simulink model "torch_pos_with_sensors_tuning(1)"  (R2024a)
settings: Solver=FixedStepAuto  StartTime=0.0  StopTime=50  FixedStep=framePeriod_s  RelTol=1e-3
undefined symbols (not defined in the file): Aircraft, DiscIntNeverNeededParam, framePeriod_s, frameRate_hz, magnitude
libraries: simulink x37, slpidlib x10, simulink_extras x2, dspmathops x1
(part 2 of 4)

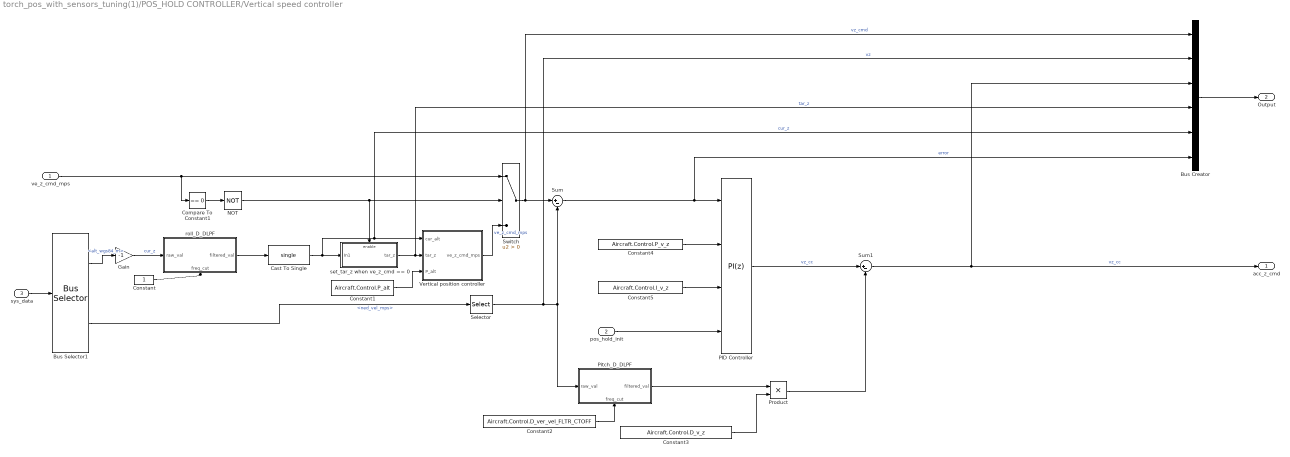
== system torch_pos_with_sensors_tuning(1)/POS_HOLD CONTROLLER/Vertical speed controller ==
  ve_z_cmd_mps : Inport
  pos_hold_init : Inport  Port=2
  sys_data : Inport  Port=3
  Bus Creator : BusCreator  Inputs=6
  Bus Selector1 : BusSelector  OutputSignals=Sensor Data.ext_gnss1.alt_wgs84_m,StateEstData.bfs_ins.ned_vel_mps
  Cast To Single : DataTypeConversion  OutDataTypeStr=single  SaturateOnIntegerOverflow=off  RndMeth=Floor
  Compare To Constant1 : simulink/Logic and Bit Operations/Compare To Constant  relop===  const=0  OutDataTypeStr=boolean
  Constant : Constant  OutDataTypeStr=single
  Constant1 : Constant  Value=Aircraft.Control.P_alt  OutDataTypeStr=single
  Constant2 : Constant  Value=Aircraft.Control.D_ver_vel_FLTR_CTOFF  OutDataTypeStr=single
  Constant3 : Constant  Value=Aircraft.Control.D_v_z  OutDataTypeStr=single
  Constant4 : Constant  Value=Aircraft.Control.P_v_z  OutDataTypeStr=single
  Constant5 : Constant  Value=Aircraft.Control.I_v_z  OutDataTypeStr=single
  Gain : Gain  Gain=-1
  NOT : Logic  Operator=NOT  IconShape=distinctive  AllPortsSameDT=off  OutDataTypeStr=boolean
  PID Controller : slpidlib/PID Controller  Controller=PI  Form=Parallel  TimeDomain=Discrete-time  UseExternalTs=off  SampleTime=framePeriod_s  IntegratorMethod=Forward Euler  FilterMethod=Forward Euler  ControllerParametersSource=external  P=0  I=0  UseKiTs=off  D=0  UseExternalDerivativeSource=off  N=100  UseFilter=off  TunerSelectOption=Frequency Response Based  InitialConditionSource=internal  InitialConditionForIntegrator=0  InitialConditionForFilter=0  DifferentiatorICPrevScaledInput=0  ExternalReset=either  TrackingMode=off  Kt=1  LimitOutput=on  SatLimitsSource=internal  UpperSaturationLimit=1  LowerSaturationLimit=-1  LinearizeAsGain=on  AntiWindupMode=clamping  Kb=1  LimitIntegrator=off  UpperIntegratorSaturationLimit=inf  LowerIntegratorSaturationLimit=-inf  POutMin=[]  POutMax=[]  IOutMin=[]  IOutMax=[]  DOutMin=[]  DOutMax=[]  NOutMin=[]  NOutMax=[]  SumOutMin=[]  SumOutMax=[]  SaturationOutMin=[]  SaturationOutMax=[]  PParamMin=[]  PParamMax=[]  IParamMin=[]  IParamMax=[]  DParamMin=[]  DParamMax=[]  NParamMin=[]  NParamMax=[]  KbParamMin=[]  KbParamMax=[]  KtParamMin=[]  KtParamMax=[]  KbOutMin=[]  KbOutMax=[]  KtOutMin=[]  KtOutMax=[]  IntegratorOutMin=[]  IntegratorOutMax=[]  FilterOutMin=[]  FilterOutMax=[]  SumI1OutMin=[]  SumI1OutMax=[]  SumI2OutMin=[]  SumI2OutMax=[]  SumI3OutMin=[]  SumI3OutMax=[]  SumI4OutMin=[]  SumI4OutMax=[]  SumDOutMin=[]  SumDOutMax=[]  DifferentiatorOutMin=[]  DifferentiatorOutMax=[]  FilterDiffOutCoefMin=[]  FilterDiffOutCoefMax=[]  ReciprocalOutMin=[]  ReciprocalOutMax=[]  SumDenOutMin=[]  SumDenOutMax=[]  SumNumOutMin=[]  SumNumOutMax=[]  DivideOutMin=[]  DivideOutMax=[]  UdiffTsProdOutMin=[]  UdiffTsProdOutMax=[]  NTsProdOutMin=[]  NTsProdOutMax=[]  UintegralTsProdOutMin=[]  UintegralTsProdOutMax=[]  UngainTsProdOutMin=[]  UngainTsProdOutMax=[]  ClampingZeroOutDataTypeStr=Inherit: Inherit via back propagation  ClampingZeroOutMin=[]  ClampingZeroOutMax=[]  FilterDenConstantOutDataTypeStr=Inherit: Inherit via back propagation  FilterDenConstantOutMin=[]  FilterDenConstantOutMax=[]  PCopyOutDataTypeStr=Inherit: Inherit via back propagation  PCopyOutMin=[]  PCopyOutMax=[]  NCopyOutDataTypeStr=Inherit: Inherit via back propagation  NCopyOutMin=[]  NCopyOutMax=[]  IntegratorContinuousStateAttributes=''  IntegratorStateMustResolveToSignalObject=off  IntegratorRTWStateStorageClass=Auto  FilterContinuousStateAttributes=''  FilterStateMustResolveToSignalObject=off  FilterRTWStateStorageClass=Auto  ParallelPVariant=ExternalParameters  IdealPVariant=Disabled  IVariant=ExternalParameters  DVariant=Disabled  IntegratorVariant=Discrete  SatVariant=Enabled  AWVariant=DiscClampingParallel  PCopyVariant=Disabled  TRVariant=Disabled  FdbkBlocksVariant=Forward  IdealPFdbkVariant=Disabled  SatFdbkVariant=Disabled  DerivativeFilterVariant=Disabled  NVariant=Disabled  NCopyVariant=Disabled_SignalSpec  FilterICVariant=Disabled  IntegratorICVariant=InternalICs  ExternalResetVariant=ExternalReset  TRSumVariant=Passthrough  SumFdbkVariant=Disabled  SumVariant=Sum_PI  TsampFilterVariant=InternalTs  TsampNgainVariant=Passthrough  TsampIntegralVariant=Disabled_SignalSpec  ExternalSaturationOutDataTypeStr=Inherit: Same as second input  DerivativeSourceVariant=Disabled
  Pitch_D_DLPF : Subsystem
      settings: PortSchema="{\"entries\":[{\"content\":{\"sides\":[{\"content\":{\"connectorIds\":[\"In1\"]},\"type\":\"ConnectorPlacement.EquallySpacedRectSide\",\"uuid\":\"20236834-aeb3-4c5b-bb2e-f84447e752b5\"},{\"content\":{\"connectorIds\":[\"Out1\"],\"side\":\"RIGHT\"},\"type\":\"ConnectorPlacement.EquallySpacedRectSide\",\"uuid\":\"d668f9a1-a3df-4207-8bf1-99fb838e59b2\"},{\"content\":{\"connectorIds\":[],\"side\":\"TOP\"},\"type\":\"ConnectorPlacement.EquallySpacedRectSide\",\"uuid\":\"66cceb06-f4bc-4278-b965-2427292e46df\"},{\"content\":{\"connectorIds\":[\"In2\"],\"side\":\"BOTTOM\"},\"type\":\"ConnectorPlacement.EquallySpacedRectSide\",\"uuid\":\"7d08bc25-8e2d-44c6-8f94-b04e75c70268\"}]},\"type\":\"ConnectorPlacement.EquallySpacedConnector\",\"uuid\":\"3dc29a9a-e794-478d-b7df-452e6c2d3f66\"}],\"packageUris\":[\"http://schema.mathworks.com/mf0/Connector/R2020b\"],\"version\":\"1.0\"}"
  Product : Product
  Selector : Selector  InputPortWidth=3  IndexOptions=Index vector (dialog)  Indices=[3]  OutputSizes=1
  Sum : Sum  Inputs=|+-
  Sum1 : Sum  Inputs=|+-
  Switch : Switch  Criteria=u2 > Threshold  SaturateOnIntegerOverflow=off  InputSameDT=off
  Vertical position controller : Subsystem
  roll_D_DLPF : Subsystem
      settings: PortSchema="{\"entries\":[{\"content\":{\"sides\":[{\"content\":{\"connectorIds\":[\"In1\"]},\"type\":\"ConnectorPlacement.EquallySpacedRectSide\",\"uuid\":\"20236834-aeb3-4c5b-bb2e-f84447e752b5\"},{\"content\":{\"connectorIds\":[\"Out1\"],\"side\":\"RIGHT\"},\"type\":\"ConnectorPlacement.EquallySpacedRectSide\",\"uuid\":\"d668f9a1-a3df-4207-8bf1-99fb838e59b2\"},{\"content\":{\"connectorIds\":[],\"side\":\"TOP\"},\"type\":\"ConnectorPlacement.EquallySpacedRectSide\",\"uuid\":\"66cceb06-f4bc-4278-b965-2427292e46df\"},{\"content\":{\"connectorIds\":[\"In2\"],\"side\":\"BOTTOM\"},\"type\":\"ConnectorPlacement.EquallySpacedRectSide\",\"uuid\":\"8fdaac6a-cb03-4bd4-87bb-7bafd10bc297\"}]},\"type\":\"ConnectorPlacement.EquallySpacedConnector\",\"uuid\":\"3dc29a9a-e794-478d-b7df-452e6c2d3f66\"}],\"packageUris\":[\"http://schema.mathworks.com/mf0/Connector/R2020b\"],\"version\":\"1.0\"}"
  set_tar_z when ve_z_cmd == 0 : Subsystem  TreatAsAtomicUnit=on
  acc_z_cmd : Outport
  Output : Outport  Port=2
  wires:
  Constant4/1 -> PID Controller/2
  Bus Selector1/2 -> Selector/1  "<ned_vel_mps>"
  sys_data/1 -> Bus Selector1/1
  Pitch_D_DLPF/1(filtered_val) -> Product/1
  Selector/1 -> Bus Creator/2, Sum/2, Pitch_D_DLPF/1(raw_val)  "vz"
  Constant3/1 -> Product/2
  Product/1 -> Sum1/2
  ve_z_cmd_mps/1 -> Compare To Constant1/1, Switch/1
  Compare To Constant1/1 -> NOT/1
  Switch/1 -> Bus Creator/1, Sum/1  "vz_cmd"
  set_tar_z when ve_z_cmd == 0/1(tar_z) -> Bus Creator/4, Vertical position controller/2(tar_z)  "tar_z"
  pos_hold_init/1 -> PID Controller/4
  Constant2/1 -> Pitch_D_DLPF/2(freq_cut)
  Constant1/1 -> Vertical position controller/3(P_alt)
  Bus Creator/1 -> Output/1
  Cast To Single/1 -> Bus Creator/5, Vertical position controller/1(cur_alt), set_tar_z when ve_z_cmd == 0/1(In1)  "cur_z"
  Sum/1 -> Bus Creator/6, PID Controller/1  "error"
  Sum1/1 -> acc_z_cmd/1, Bus Creator/3  "vz_cc"
  PID Controller/1 -> Sum1/1  "vz_cc"
  Constant5/1 -> PID Controller/3
  Vertical position controller/1(ve_z_cmd_mps) -> Switch/3  "ve_z_cmd_mps"
  NOT/1 -> Switch/2, set_tar_z when ve_z_cmd == 0/Enable
  Bus Selector1/1 -> Gain/1  "<alt_wgs84_m>"
  Gain/1 -> roll_D_DLPF/1(raw_val)  "cur_z"
  roll_D_DLPF/1(filtered_val) -> Cast To Single/1
  Constant/1 -> roll_D_DLPF/2(freq_cut)

== system torch_pos_with_sensors_tuning(1)/Stab_input_conversion/remap from min_spin to max ==
  raw_in : Inport
  Constant4 : Constant  Value=0  OutDataTypeStr=single
  Constant5 : Constant  Value=Aircraft.Control.motor_spin_min  OutDataTypeStr=single
  Constant6 : Constant  Value=0.8  OutDataTypeStr=single
  Constant7 : Constant  OutDataTypeStr=single
  remap1 : MATLAB Function  TreatAsAtomicUnit=on
  norm_out : Outport
  wires:
  Constant6/1 -> remap1/5(out_max)
  Constant5/1 -> remap1/4(out_min)
  remap1/1(norm_out) -> norm_out/1
  Constant4/1 -> remap1/2(in_min)
  Constant7/1 -> remap1/3(in_max)
  raw_in/1 -> remap1/1(raw_in)

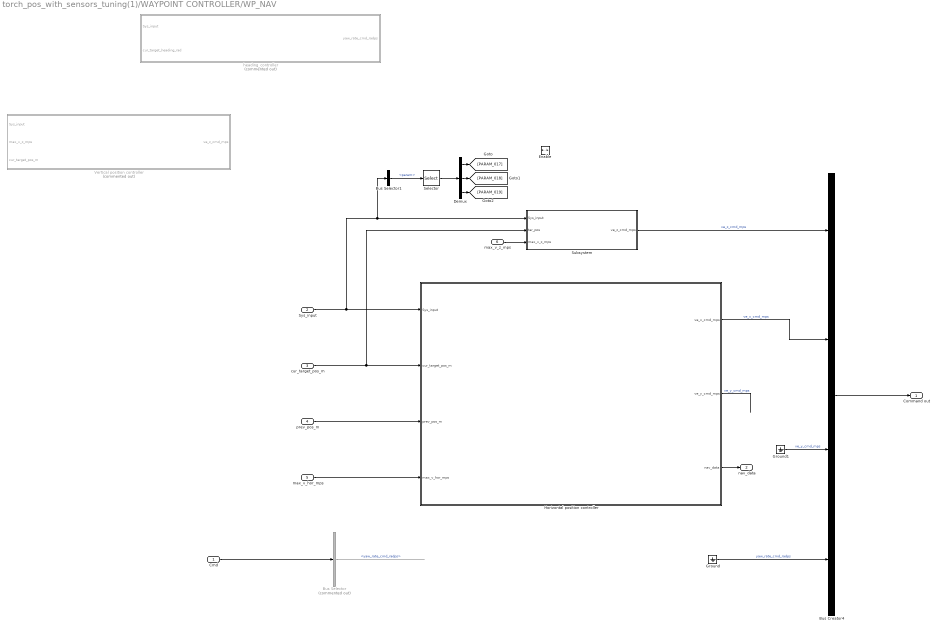
== system torch_pos_with_sensors_tuning(1)/WAYPOINT CONTROLLER/WP_NAV ==
  Cmd : Inport
  Sys_input : Inport  Port=2
  cur_target_pos_m : Inport  Port=3
  prev_pos_m : Inport  Port=4
  max_v_hor_mps : Inport  Port=5
  max_v_z_mps : Inport  Port=6
  Enable : EnablePort
  Bus Creator4 : BusCreator  Inputs=4
  Bus Selector : BusSelector  Commented=on  OutputSignals=yaw_rate_cmd_radps
  Bus Selector1 : BusSelector  OutputSignals=Telemetry Data.param
  Demux : Demux  Outputs=3
  Ground : Ground
  Ground1 : Ground
  Horizontal position controller : Subsystem
  Selector : Selector  IndexMode=Zero-based  InputPortWidth=24  IndexOptions=Index vector (dialog)  Indices=[17 18 19]  OutputSizes=1
  Subsystem : Subsystem
  Vertical position controller : Subsystem  Commented=on
  heading_controller : Subsystem  Commented=on
  Command out : Outport
  nav_data : Outport  Port=2
  wires:
  Bus Creator4/1 -> Command out/1
  Horizontal position controller/1(ve_x_cmd_mps) -> Bus Creator4/2  "ve_x_cmd_mps"
  Horizontal position controller/2(ve_y_cmd_mps) -> ?  "ve_y_cmd_mps"
  Sys_input/1 -> Horizontal position controller/1(Sys_input), Bus Selector1/1, Subsystem/1(Sys_input)
  cur_target_pos_m/1 -> Subsystem/2(tar_pos), Horizontal position controller/2(cur_target_pos_m)
  Cmd/1 -> Bus Selector/1
  Bus Selector/1 -> ?  "<yaw_rate_cmd_radps>"
  prev_pos_m/1 -> Horizontal position controller/3(prev_pos_m)
  max_v_hor_mps/1 -> Horizontal position controller/4(max_v_hor_mps)
  Subsystem/1(ve_z_cmd_mps) -> Bus Creator4/1  "ve_z_cmd_mps"
  max_v_z_mps/1 -> Subsystem/3(max_v_z_mps)
  Horizontal position controller/3(nav_data) -> nav_data/1
  Ground/1 -> Bus Creator4/4  "yaw_rate_cmd_radps"
  Ground1/1 -> Bus Creator4/3  "ve_y_cmd_mps"
  Selector/1 -> Demux/1
  Demux/1 -> [PARAM_017]
  Demux/2 -> [PARAM_018]
  Demux/3 -> [PARAM_019]
  Bus Selector1/1 -> Selector/1  "<param>"

== system torch_pos_with_sensors_tuning(1)/WAYPOINT CONTROLLER/capture rising edge ==
  <current_waypoint> : Inport
  Detect Change1 : simulink/Logic and Bit Operations/Detect Change  vinit=-1  OutDataTypeStr=boolean
  Detect Rise Positive : simulink/Logic and Bit Operations/Detect Rise Positive  Commented=through  vinit=0  OutDataTypeStr=boolean
  enable : Outport
  wires:
  <current_waypoint>/1 -> Detect Change1/1
  Detect Rise Positive/1 -> enable/1
  Detect Change1/1 -> Detect Rise Positive/1

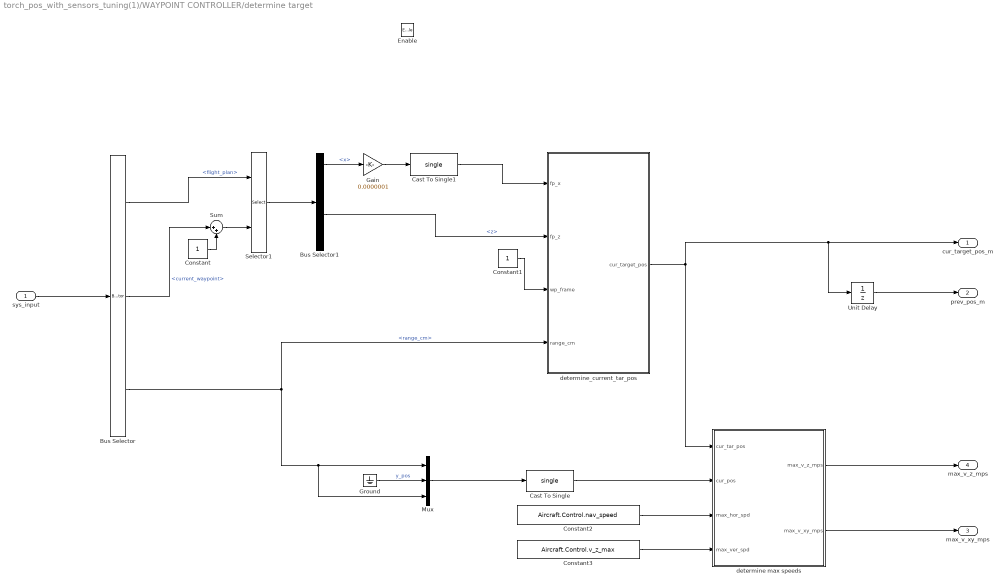
== system torch_pos_with_sensors_tuning(1)/WAYPOINT CONTROLLER/determine target ==
  sys_input : Inport
  Enable : EnablePort  PropagateVarSize=During execution
  Bus Selector : BusSelector  OutputSignals=Telemetry Data.flight_plan,Telemetry Data.current_waypoint,Sensor Data.tfmini.range_cm
  Bus Selector1 : BusSelector  OutputSignals=x,y,z,frame
  Cast To Single : DataTypeConversion  OutDataTypeStr=single  SaturateOnIntegerOverflow=off  RndMeth=Floor
  Cast To Single1 : DataTypeConversion  OutDataTypeStr=single  SaturateOnIntegerOverflow=off  RndMeth=Floor
  Constant : Constant  OutDataTypeStr=int16
  Constant1 : Constant  OutDataTypeStr=uint8
  Constant2 : Constant  Value=Aircraft.Control.nav_speed  OutDataTypeStr=single
  Constant3 : Constant  Value=Aircraft.Control.v_z_max  OutDataTypeStr=single
  Gain : Gain  Gain=0.0000001  OutDataTypeStr=double
  Ground : Ground
  Mux : Mux  Inputs=3
  Selector1 : Selector  IndexMode=Zero-based  InputPortWidth=500  IndexOptions=Index vector (port)  Indices=[1 3]  OutputSizes=1
  Sum : Sum  Inputs=|++
  Unit Delay : UnitDelay  InitialCondition=[0 0 0]  SampleTime=-1  HasFrameUpgradeWarning=on
  determine max speeds : MATLAB Function  TreatAsAtomicUnit=on
  determine_current_tar_pos : MATLAB Function  TreatAsAtomicUnit=on
  cur_target_pos_m : Outport
  prev_pos_m : Outport  Port=2
  max_v_xy_mps : Outport  Port=3
  max_v_z_mps : Outport  Port=4
  wires:
  sys_input/1 -> Bus Selector/1
  Selector1/1 -> Bus Selector1/1
  Bus Selector1/3 -> determine_current_tar_pos/2(fp_z)  "<z>"
  Bus Selector1/1 -> Gain/1  "<x>"
  Bus Selector/1 -> Selector1/1  "<flight_plan>"
  Gain/1 -> Cast To Single1/1
  Sum/1 -> Selector1/2
  Constant/1 -> Sum/2
  Constant1/1 -> determine_current_tar_pos/3(wp_frame)
  Unit Delay/1 -> prev_pos_m/1
  determine_current_tar_pos/1(cur_target_pos) -> cur_target_pos_m/1, Unit Delay/1, determine max speeds/1(cur_tar_pos)
  Cast To Single1/1 -> determine_current_tar_pos/1(fp_x)
  Constant2/1 -> determine max speeds/3(max_hor_spd)
  Constant3/1 -> determine max speeds/4(max_ver_spd)
  determine max speeds/1(max_v_z_mps) -> max_v_z_mps/1
  determine max speeds/2(max_v_xy_mps) -> max_v_xy_mps/1
  Bus Selector/3 -> Mux/3, Mux/1, determine_current_tar_pos/4(range_cm)  "<range_cm>"
  Bus Selector/2 -> Sum/1  "<current_waypoint>"
  Mux/1 -> Cast To Single/1
  Ground/1 -> Mux/2  "y_pos"
  Cast To Single/1 -> determine max speeds/2(cur_pos)

== system torch_pos_with_sensors_tuning(1)/WAYPOINT CONTROLLER/wp_completion_check ==
  note: Output wp_reached cmd only when distance between current pos and target pos is less than wp_radius.
  target_pos : Inport
  Sys_input : Inport  Port=2
  Bus Selector : BusSelector  OutputSignals=Sensor Data.tfmini.range_cm
  Constant : Constant  Value=Aircraft.Control.wp_radius  OutDataTypeStr=single
  check_wp_reached : MATLAB Function  TreatAsAtomicUnit=on
  wp_reached : Outport
  wires:
  Sys_input/1 -> Bus Selector/1
  Bus Selector/1 -> check_wp_reached/2(range_cm)  "<range_cm>"
  check_wp_reached/1(reached) -> wp_reached/1
  target_pos/1 -> check_wp_reached/1(target_pos)
  Constant/1 -> check_wp_reached/3(Aircraft_Control_wp_radius)

== system torch_pos_with_sensors_tuning(1)/WAYPOINT CONTROLLER CMD/Throttle Mapper ==
  Throttle : Inport
  Compare To Constant : simulink/Logic and Bit Operations/Compare To Constant  relop=<  const=0  OutDataTypeStr=boolean
  Compare To Constant1 : simulink/Logic and Bit Operations/Compare To Constant  relop=>=  const=0  OutDataTypeStr=boolean
  Constant : Constant  Value=Aircraft.Control.v_z_down_max  OutDataTypeStr=single
  Constant1 : Constant  Value=Aircraft.Control.v_z_up_max  OutDataTypeStr=single
  Double : Constant  Value=2  OutDataTypeStr=single
  Gain : Gain  Gain=-1
  Normalize at Zero : Constant  Value=0.5  OutDataTypeStr=single
  Product : Product  Inputs=3
  Product1 : Product  Inputs=3
  Sum : Sum  Inputs=|+-
  Sum1 : Sum
  v_z_cmd (-1 to 1) : Product
  Relative Velocity : Outport
  wires:
  Throttle/1 -> Sum/1
  Normalize at Zero/1 -> Sum/2
  Double/1 -> v_z_cmd (-1 to 1)/2
  Sum/1 -> v_z_cmd (-1 to 1)/1
  Sum1/1 -> Gain/1
  v_z_cmd (-1 to 1)/1 -> Product1/2, Compare To Constant1/1, Compare To Constant/1, Product/3
  Constant1/1 -> Product1/3
  Compare To Constant1/1 -> Product1/1
  Product/1 -> Sum1/1
  Product1/1 -> Sum1/2
  Constant/1 -> Product/1
  Compare To Constant/1 -> Product/2
  Gain/1 -> Relative Velocity/1

== system torch_pos_with_sensors_tuning(1)/WAYPOINT CONTROLLER CMD/pitch_norm_deadband ==
  raw_sbus_in : Inport
  deadband : Inport  Port=2
  Constant : Constant  Value=0  OutDataTypeStr=single
  Constant1 : Constant  Value=0  OutDataTypeStr=single
  Constant2 : Constant  OutDataTypeStr=single
  Constant3 : Constant  OutDataTypeStr=single
  remap_with_deadband : MATLAB Function  TreatAsAtomicUnit=on
  normalized_out : Outport
  wires:
  deadband/1 -> remap_with_deadband/6(deadband)
  Constant2/1 -> remap_with_deadband/5(out_max)
  Constant1/1 -> remap_with_deadband/4(out_min)
  Constant3/1 -> remap_with_deadband/3(in_max)
  Constant/1 -> remap_with_deadband/2(in_min)
  remap_with_deadband/1(norm_out) -> normalized_out/1
  raw_sbus_in/1 -> remap_with_deadband/1(raw_in)

== system torch_pos_with_sensors_tuning(1)/WAYPOINT CONTROLLER CMD/remap from min_spin to max ==
  raw_in : Inport
  Constant4 : Constant  Value=0  OutDataTypeStr=single
  Constant5 : Constant  Value=Aircraft.Control.motor_spin_min  OutDataTypeStr=single
  Constant6 : Constant  OutDataTypeStr=single
  Constant7 : Constant  OutDataTypeStr=single
  remap1 : MATLAB Function  TreatAsAtomicUnit=on
  norm_out : Outport
  wires:
  Constant6/1 -> remap1/5(out_max)
  Constant5/1 -> remap1/4(out_min)
  remap1/1(norm_out) -> norm_out/1
  Constant4/1 -> remap1/2(in_min)
  Constant7/1 -> remap1/3(in_max)
  raw_in/1 -> remap1/1(raw_in)

== system torch_pos_with_sensors_tuning(1)/cmd to raw pwm1/motor_PWM_denormalize ==
  normalized_input : Inport
  Constant : Constant  Value=0  OutDataTypeStr=single
  Constant1 : Constant  Value=1100  OutDataTypeStr=single
  Constant2 : Constant  Value=1950  OutDataTypeStr=single
  Constant3 : Constant  OutDataTypeStr=single
  remap : MATLAB Function  TreatAsAtomicUnit=on
  raw_output : Outport
  wires:
  Constant2/1 -> remap/5(out_max)
  Constant1/1 -> remap/4(out_min)
  Constant3/1 -> remap/3(in_max)
  Constant/1 -> remap/2(in_min)
  remap/1(raw_out) -> raw_output/1
  normalized_input/1 -> remap/1(norm_in)

== system torch_pos_with_sensors_tuning(1)/command selection/e_stop_norm ==
  raw_sbus_in : Inport
  Constant : Constant  Value=172  OutDataTypeStr=single
  Constant1 : Constant  Value=-1  OutDataTypeStr=single
  Constant2 : Constant  OutDataTypeStr=single
  Constant3 : Constant  Value=1811  OutDataTypeStr=single
  remap : MATLAB Function  TreatAsAtomicUnit=on
  normalized_out : Outport
  wires:
  Constant2/1 -> remap/5(out_max)
  Constant1/1 -> remap/4(out_min)
  Constant3/1 -> remap/3(in_max)
  Constant/1 -> remap/2(in_min)
  remap/1(norm_out) -> normalized_out/1
  raw_sbus_in/1 -> remap/1(raw_in)

== system torch_pos_with_sensors_tuning(1)/command selection/mode_norm ==
  raw_sbus_in : Inport
  Constant : Constant  Value=172  OutDataTypeStr=single
  Constant1 : Constant  Value=0  OutDataTypeStr=single
  Constant2 : Constant  Value=2  OutDataTypeStr=single
  Constant3 : Constant  Value=1811  OutDataTypeStr=single
  remap : MATLAB Function  TreatAsAtomicUnit=on
  normalized_out : Outport
  wires:
  raw_sbus_in/1 -> remap/1(raw_in)
  remap/1(norm_out) -> normalized_out/1
  Constant/1 -> remap/2(in_min)
  Constant3/1 -> remap/3(in_max)
  Constant1/1 -> remap/4(out_min)
  Constant2/1 -> remap/5(out_max)

== system torch_pos_with_sensors_tuning(1)/command selection/mode_norm1 ==
  raw_sbus_in : Inport
  Constant : Constant  Value=172  OutDataTypeStr=single
  Constant1 : Constant  Value=0  OutDataTypeStr=single
  Constant2 : Constant  OutDataTypeStr=single
  Constant3 : Constant  Value=1811  OutDataTypeStr=single
  remap : MATLAB Function  TreatAsAtomicUnit=on
  normalized_out : Outport
  wires:
  Constant2/1 -> remap/5(out_max)
  Constant1/1 -> remap/4(out_min)
  Constant3/1 -> remap/3(in_max)
  Constant/1 -> remap/2(in_min)
  remap/1(norm_out) -> normalized_out/1
  raw_sbus_in/1 -> remap/1(raw_in)

== system torch_pos_with_sensors_tuning(1)/command selection/pitch_norm_deadband ==
  raw_sbus_in : Inport
  deadband : Inport  Port=2
  Constant : Constant  Value=172  OutDataTypeStr=single
  Constant1 : Constant  Value=-1  OutDataTypeStr=single
  Constant2 : Constant  OutDataTypeStr=single
  Constant3 : Constant  Value=1811  OutDataTypeStr=single
  remap_with_deadband : MATLAB Function  TreatAsAtomicUnit=on
  normalized_out : Outport
  wires:
  deadband/1 -> remap_with_deadband/6(deadband)
  Constant2/1 -> remap_with_deadband/5(out_max)
  Constant1/1 -> remap_with_deadband/4(out_min)
  Constant3/1 -> remap_with_deadband/3(in_max)
  Constant/1 -> remap_with_deadband/2(in_min)
  remap_with_deadband/1(norm_out) -> normalized_out/1
  raw_sbus_in/1 -> remap_with_deadband/1(raw_in)

== system torch_pos_with_sensors_tuning(1)/command selection/roll_norm_deadband ==
  raw_sbus_in : Inport
  deadband : Inport  Port=2
  Constant : Constant  Value=172  OutDataTypeStr=single
  Constant1 : Constant  Value=-1  OutDataTypeStr=single
  Constant2 : Constant  OutDataTypeStr=single
  Constant3 : Constant  Value=1811  OutDataTypeStr=single
  remap_with_deadband : MATLAB Function  TreatAsAtomicUnit=on
  normalized_out : Outport
  wires:
  deadband/1 -> remap_with_deadband/6(deadband)
  Constant2/1 -> remap_with_deadband/5(out_max)
  Constant1/1 -> remap_with_deadband/4(out_min)
  Constant3/1 -> remap_with_deadband/3(in_max)
  Constant/1 -> remap_with_deadband/2(in_min)
  remap_with_deadband/1(norm_out) -> normalized_out/1
  raw_sbus_in/1 -> remap_with_deadband/1(raw_in)

== system torch_pos_with_sensors_tuning(1)/command selection/throttle_norm ==
  raw_sbus_in : Inport
  Constant : Constant  Value=172  OutDataTypeStr=single
  Constant1 : Constant  Value=0  OutDataTypeStr=single
  Constant2 : Constant  OutDataTypeStr=single
  Constant3 : Constant  Value=1811  OutDataTypeStr=single
  remap : MATLAB Function  TreatAsAtomicUnit=on
  normalized_out : Outport
  wires:
  raw_sbus_in/1 -> remap/1(raw_in)
  remap/1(norm_out) -> normalized_out/1
  Constant/1 -> remap/2(in_min)
  Constant3/1 -> remap/3(in_max)
  Constant1/1 -> remap/4(out_min)
  Constant2/1 -> remap/5(out_max)

== system torch_pos_with_sensors_tuning(1)/command selection/yaw_norm_deadband ==
  raw_sbus_in : Inport
  deadband : Inport  Port=2
  Constant : Constant  Value=172  OutDataTypeStr=single
  Constant1 : Constant  Value=-1  OutDataTypeStr=single
  Constant2 : Constant  OutDataTypeStr=single
  Constant3 : Constant  Value=1811  OutDataTypeStr=single
  remap_with_deadband : MATLAB Function  TreatAsAtomicUnit=on
  normalized_out : Outport
  wires:
  raw_sbus_in/1 -> remap_with_deadband/1(raw_in)
  remap_with_deadband/1(norm_out) -> normalized_out/1
  Constant/1 -> remap_with_deadband/2(in_min)
  Constant3/1 -> remap_with_deadband/3(in_max)
  Constant1/1 -> remap_with_deadband/4(out_min)
  Constant2/1 -> remap_with_deadband/5(out_max)
  deadband/1 -> remap_with_deadband/6(deadband)

== system torch_pos_with_sensors_tuning(1)/determine arm and mode selection/Failsafe_management ==
  note: - radio failsafe
  In Bus Element1 : Inport  PortName=inceptor  Element=failsafe
  manual_mode : Inport  Port=2
  motor_state : Inport  Port=3
  NOT : Logic  Operator=NOT  IconShape=distinctive  AllPortsSameDT=off  OutDataTypeStr=boolean
  Radio failsafe : Subsystem
  radio_failsafe_enabled : Outport
  wires:
  Radio failsafe/1(radio_failsafe_enabled) -> radio_failsafe_enabled/1
  manual_mode/1 -> Radio failsafe/2(manual_mode)
  motor_state/1 -> Radio failsafe/3(motor_state)
  In Bus Element1/1 -> NOT/1
  NOT/1 -> Radio failsafe/1(failsafe)

== system torch_pos_with_sensors_tuning(1)/determine arm and mode selection/Subsystem ==
  <e_stop> : Inport
  Abs1 : Abs  SaturateOnIntegerOverflow=off
  Compare To Constant : simulink/Logic and Bit Operations/Compare To Constant  relop=>=  const=0.98  OutDataTypeStr=boolean
  e_stop counter : Subsystem
  e_stop_filtered : Outport
  wires:
  Compare To Constant/1 -> e_stop counter/Enable
  Abs1/1 -> Compare To Constant/1
  <e_stop>/1 -> e_stop counter/1(motor_e_stop_raw), Abs1/1
  e_stop counter/1(e_stop_filtered) -> e_stop_filtered/1

== system torch_pos_with_sensors_tuning(1)/determine arm and mode selection/yaw_stick_arming ==
  note: yaw_stick arming
  <yaw> : Inport
  <throttle> : Inport  Port=2
  e_stop : Inport  Port=3
  AND : Logic  IconShape=distinctive  AllPortsSameDT=off  OutDataTypeStr=boolean
  Abs : Abs  SaturateOnIntegerOverflow=off
  Cast To Single : DataTypeConversion  OutDataTypeStr=single  SaturateOnIntegerOverflow=off  RndMeth=Floor
  Compare To Constant : simulink/Logic and Bit Operations/Compare To Constant  relop=>  const=0  OutDataTypeStr=boolean
  Compare To Constant1 : simulink/Logic and Bit Operations/Compare To Constant  relop=>=  const=0.95  OutDataTypeStr=boolean
  Compare To Constant2 : simulink/Logic and Bit Operations/Compare To Constant  relop=>=  const=3  OutDataTypeStr=boolean
  Compare To Constant3 : simulink/Logic and Bit Operations/Compare To Constant  relop=<=  const=0.03  OutDataTypeStr=boolean
  Compare To Constant4 : simulink/Logic and Bit Operations/Compare To Constant  relop=>=  const=0.5  OutDataTypeStr=boolean
  Constant : Constant  Value=0  OutDataTypeStr=boolean  LockScale=on
  Enabled Subsystem : Subsystem  TreatAsAtomicUnit=on
  OR : Logic  Operator=OR  IconShape=distinctive  AllPortsSameDT=off  OutDataTypeStr=boolean
  Sum : Sum  Inputs=-+|
  Switch : Switch  Criteria=u2 > Threshold  SaturateOnIntegerOverflow=off  InputSameDT=off
  Unit Delay : UnitDelay  SampleTime=-1  HasFrameUpgradeWarning=on
  manual_arming : Subsystem
  arm_state : Outport
  wires:
  Enabled Subsystem/1(time_arm_valid_s) -> Compare To Constant2/1
  Abs/1 -> Compare To Constant1/1
  Compare To Constant1/1 -> AND/2, Enabled Subsystem/1(yaw_input)
  Compare To Constant4/1 -> manual_arming/1(yaw_arm)
  AND/1 -> Enabled Subsystem/Enable
  <yaw>/1 -> Compare To Constant4/1, Abs/1
  <throttle>/1 -> Compare To Constant3/1
  Compare To Constant3/1 -> AND/1
  Constant/1 -> Switch/1
  manual_arming/1(arm_state) -> Switch/3
  Switch/1 -> arm_state/1
  e_stop/1 -> OR/1, Switch/2
  OR/1 -> manual_arming/Trigger
  Compare To Constant2/1 -> Cast To Single/1
  Sum/1 -> Compare To Constant/1
  Unit Delay/1 -> Sum/1
  Cast To Single/1 -> Unit Delay/1, Sum/2
  Compare To Constant/1 -> OR/2

== system torch_pos_with_sensors_tuning(1)/ANGLE CONTROLLER1/Pitch Controller/pitch_D_DLPF ==
  raw_val : Inport
  freq_cut : Inport  Port=2
  Constant : Constant  Value=frameRate_hz  OutDataTypeStr=single
  MATLAB Function : MATLAB Function  TreatAsAtomicUnit=on
  Unit Delay : UnitDelay  SampleTime=-1  HasFrameUpgradeWarning=on
  filtered_val : Outport
  wires:
  freq_cut/1 -> MATLAB Function/3(freq_cut)
  MATLAB Function/1(filtered_val) -> Unit Delay/1, filtered_val/1
  Unit Delay/1 -> MATLAB Function/1(prev_val)
  raw_val/1 -> MATLAB Function/2(raw_val)
  Constant/1 -> MATLAB Function/4(samp_freq)

== system torch_pos_with_sensors_tuning(1)/ANGLE CONTROLLER1/Pitch Controller/pitch_input_DLPF ==
  raw_val : Inport
  freq_cut : Inport  Port=2
  Constant : Constant  Value=frameRate_hz  OutDataTypeStr=single
  MATLAB Function : MATLAB Function  TreatAsAtomicUnit=on
  Unit Delay : UnitDelay  SampleTime=-1  HasFrameUpgradeWarning=on
  filtered_val : Outport
  wires:
  Constant/1 -> MATLAB Function/4(samp_freq)
  raw_val/1 -> MATLAB Function/2(raw_val)
  Unit Delay/1 -> MATLAB Function/1(prev_val)
  MATLAB Function/1(filtered_val) -> filtered_val/1, Unit Delay/1
  freq_cut/1 -> MATLAB Function/3(freq_cut)

== system torch_pos_with_sensors_tuning(1)/POS_HOLD CONTROLLER/Horizontal speed controller/Subsystem ==
  ve_x cmd : Inport
  ve_x : Inport  Port=2
  pos_hold_init : Inport  Port=3
  Acc_x_PID : slpidlib/PID Controller  Controller=PI  Form=Parallel  TimeDomain=Discrete-time  UseExternalTs=off  SampleTime=framePeriod_s  IntegratorMethod=Forward Euler  FilterMethod=Forward Euler  ControllerParametersSource=external  P=0.335  I=0.005  UseKiTs=off  D=0  UseExternalDerivativeSource=off  N=100  UseFilter=off  TunerSelectOption=Transfer Function Based (PID Tuner App)  InitialConditionSource=internal  InitialConditionForIntegrator=0  InitialConditionForFilter=0  DifferentiatorICPrevScaledInput=0  ExternalReset=either  TrackingMode=off  Kt=1  LimitOutput=off  SatLimitsSource=internal  UpperSaturationLimit=Aircraft.Control.pitch_angle_lim  LowerSaturationLimit=-Aircraft.Control.pitch_angle_lim  LinearizeAsGain=off  AntiWindupMode=clamping  Kb=1  LimitIntegrator=off  UpperIntegratorSaturationLimit=inf  LowerIntegratorSaturationLimit=-inf  POutMin=[]  POutMax=[]  IOutMin=[]  IOutMax=[]  DOutMin=[]  DOutMax=[]  NOutMin=[]  NOutMax=[]  SumOutMin=[]  SumOutMax=[]  SaturationOutMin=[]  SaturationOutMax=[]  PParamMin=[]  PParamMax=[]  IParamMin=[]  IParamMax=[]  DParamMin=[]  DParamMax=[]  NParamMin=[]  NParamMax=[]  KbParamMin=[]  KbParamMax=[]  KtParamMin=[]  KtParamMax=[]  KbOutMin=[]  KbOutMax=[]  KtOutMin=[]  KtOutMax=[]  IntegratorOutMin=[]  IntegratorOutMax=[]  FilterOutMin=[]  FilterOutMax=[]  SumI1OutMin=[]  SumI1OutMax=[]  SumI2OutMin=[]  SumI2OutMax=[]  SumI3OutMin=[]  SumI3OutMax=[]  SumI4OutMin=[]  SumI4OutMax=[]  SumDOutMin=[]  SumDOutMax=[]  DifferentiatorOutMin=[]  DifferentiatorOutMax=[]  FilterDiffOutCoefMin=[]  FilterDiffOutCoefMax=[]  ReciprocalOutMin=[]  ReciprocalOutMax=[]  SumDenOutMin=[]  SumDenOutMax=[]  SumNumOutMin=[]  SumNumOutMax=[]  DivideOutMin=[]  DivideOutMax=[]  UdiffTsProdOutMin=[]  UdiffTsProdOutMax=[]  NTsProdOutMin=[]  NTsProdOutMax=[]  UintegralTsProdOutMin=[]  UintegralTsProdOutMax=[]  UngainTsProdOutMin=[]  UngainTsProdOutMax=[]  ClampingZeroOutDataTypeStr=Inherit: Inherit via back propagation  ClampingZeroOutMin=[]  ClampingZeroOutMax=[]  FilterDenConstantOutDataTypeStr=Inherit: Inherit via back propagation  FilterDenConstantOutMin=[]  FilterDenConstantOutMax=[]  PCopyOutDataTypeStr=Inherit: Inherit via back propagation  PCopyOutMin=[]  PCopyOutMax=[]  NCopyOutDataTypeStr=Inherit: Inherit via back propagation  NCopyOutMin=[]  NCopyOutMax=[]  IntegratorContinuousStateAttributes=''  IntegratorStateMustResolveToSignalObject=off  IntegratorRTWStateStorageClass=Auto  FilterContinuousStateAttributes=''  FilterStateMustResolveToSignalObject=off  FilterRTWStateStorageClass=Auto  ParallelPVariant=ExternalParameters  IdealPVariant=Disabled  IVariant=ExternalParameters  DVariant=Disabled  IntegratorVariant=Discrete  SatVariant=Disabled  AWVariant=Passthrough  PCopyVariant=Disabled  TRVariant=Disabled  FdbkBlocksVariant=Forward  IdealPFdbkVariant=Disabled  SatFdbkVariant=Disabled  DerivativeFilterVariant=Disabled  NVariant=Disabled  NCopyVariant=Disabled_SignalSpec  FilterICVariant=Disabled  IntegratorICVariant=InternalICs  ExternalResetVariant=ExternalReset  TRSumVariant=Passthrough  SumFdbkVariant=Disabled  SumVariant=Sum_PI  TsampFilterVariant=InternalTs  TsampNgainVariant=Passthrough  TsampIntegralVariant=Disabled_SignalSpec  ExternalSaturationOutDataTypeStr=Inherit: Same as second input  DerivativeSourceVariant=Disabled
  Bus Creator : BusCreator  Inputs=2
  Constant : Constant  Value=Aircraft.Control.FF_att_rate  OutDataTypeStr=single
  Constant1 : Constant  Value=Aircraft.Control.P_att_rate  OutDataTypeStr=single
  Constant2 : Constant  Value=Aircraft.Control.I_att_rate  OutDataTypeStr=single
  Constant3 : Constant  Value=Aircraft.Control.D_att_FLTR_CTOFF  OutDataTypeStr=single
  Constant4 : Constant  Value=Aircraft.Control.D_att_rate  OutDataTypeStr=single
  Discrete Derivative : simulink/Discrete/Discrete Derivative  gainval=1.0  ICPrevScaledInput=0.0  OutMin=[]  OutMax=[]  OutDataType=fixdt(1, 16)  OutScaling=2^-10  DoSatur=off
  Product : Product
  Product1 : Product
  Sum : Sum  Inputs=|+-
  Sum1 : Sum  Inputs=++-
  roll_D_DLPF : Subsystem
      settings: PortSchema="{\"entries\":[{\"content\":{\"sides\":[{\"content\":{\"connectorIds\":[\"In1\"]},\"type\":\"ConnectorPlacement.EquallySpacedRectSide\",\"uuid\":\"20236834-aeb3-4c5b-bb2e-f84447e752b5\"},{\"content\":{\"connectorIds\":[\"Out1\"],\"side\":\"RIGHT\"},\"type\":\"ConnectorPlacement.EquallySpacedRectSide\",\"uuid\":\"d668f9a1-a3df-4207-8bf1-99fb838e59b2\"},{\"content\":{\"connectorIds\":[],\"side\":\"TOP\"},\"type\":\"ConnectorPlacement.EquallySpacedRectSide\",\"uuid\":\"66cceb06-f4bc-4278-b965-2427292e46df\"},{\"content\":{\"connectorIds\":[\"In2\"],\"side\":\"BOTTOM\"},\"type\":\"ConnectorPlacement.EquallySpacedRectSide\",\"uuid\":\"8fdaac6a-cb03-4bd4-87bb-7bafd10bc297\"}]},\"type\":\"ConnectorPlacement.EquallySpacedConnector\",\"uuid\":\"3dc29a9a-e794-478d-b7df-452e6c2d3f66\"}],\"packageUris\":[\"http://schema.mathworks.com/mf0/Connector/R2020b\"],\"version\":\"1.0\"}"
  acc_x_cmd : Outport
  Output : Outport  Port=2
  wires:
  ve_x/1 -> Bus Creator/2, roll_D_DLPF/1(raw_val), Sum/2  "ve_x"
  Sum/1 -> Acc_x_PID/1
  Constant1/1 -> Acc_x_PID/2
  Constant2/1 -> Acc_x_PID/3  "I_gain"
  pos_hold_init/1 -> Acc_x_PID/4
  Constant4/1 -> Product/2  "D_gain"
  Discrete Derivative/1 -> Product/1
  Constant3/1 -> roll_D_DLPF/2(freq_cut)
  roll_D_DLPF/1(filtered_val) -> Discrete Derivative/1
  Bus Creator/1 -> Output/1
  ve_x cmd/1 -> Product1/2, Sum/1, Bus Creator/1  "ve_x_cmd"
  Sum1/1 -> acc_x_cmd/1
  Constant/1 -> Product1/1
  Product1/1 -> Sum1/1
  Acc_x_PID/1 -> Sum1/2
  Product/1 -> Sum1/3

== system torch_pos_with_sensors_tuning(1)/POS_HOLD CONTROLLER/Horizontal speed controller/zero_vel_handling ==
  ve_x cmd : Inport
  pos_e_feedback : Inport  Port=2
  pos_hold_init : Inport  Port=3
  Cast To Single : DataTypeConversion  OutDataTypeStr=single  SaturateOnIntegerOverflow=off  RndMeth=Floor
  Cast To Single1 : DataTypeConversion  OutDataTypeStr=single  SaturateOnIntegerOverflow=off  RndMeth=Floor
  Compare To Constant : simulink/Logic and Bit Operations/Compare To Constant  relop===  const=0  OutDataTypeStr=boolean
  Detect Change : simulink/Logic and Bit Operations/Detect Change  vinit=0  OutDataTypeStr=boolean
  Horizontal position controller : Subsystem
  Mux1 : Mux  Inputs=2
  NOT : Logic  Operator=NOT  IconShape=distinctive  AllPortsSameDT=off  OutDataTypeStr=boolean
  OR : Logic  Operator=OR  IconShape=distinctive  AllPortsSameDT=off  OutDataTypeStr=boolean
  Switch : Switch  Criteria=u2 > Threshold  SaturateOnIntegerOverflow=off  InputSameDT=off
  Unit Delay : UnitDelay  SampleTime=-1  HasFrameUpgradeWarning=on
  delay_on_instant_off : Subsystem
  set_tar_pos when vel_cmd == 0 : Subsystem  TreatAsAtomicUnit=on
  v_cmd : Outport
  Output : Outport  Port=2
  tar_get : Outport  Port=3
  wires:
  Switch/1 -> v_cmd/1
  pos_e_feedback/1 -> set_tar_pos when vel_cmd == 0/1(pos_xy_m), Horizontal position controller/2(cur_pos_m)
  set_tar_pos when vel_cmd == 0/1(target_pos_xy_m) -> Cast To Single1/1, Horizontal position controller/1(cur_target_pos_m)
  OR/1 -> delay_on_instant_off/1(in)
  Compare To Constant/1 -> OR/1
  pos_hold_init/1 -> Unit Delay/1
  Detect Change/1 -> OR/2
  Unit Delay/1 -> Detect Change/1
  Cast To Single1/1 -> Output/1
  ve_x cmd/1 -> Switch/1, Compare To Constant/1
  Horizontal position controller/1(ve_xy) -> Switch/3  "ve_xy"
  NOT/1 -> Switch/2, set_tar_pos when vel_cmd == 0/Enable
  delay_on_instant_off/1(out) -> NOT/1
  Horizontal position controller/3(bearing_to_tar) -> Mux1/2
  Mux1/1 -> Cast To Single/1
  Horizontal position controller/2(dist_to_tar) -> Mux1/1
  Cast To Single/1 -> tar_get/1

== system torch_pos_with_sensors_tuning(1)/POS_HOLD CONTROLLER/Vertical speed controller/Pitch_D_DLPF ==
  raw_val : Inport
  freq_cut : Inport  Port=2
  MATLAB Function : MATLAB Function  TreatAsAtomicUnit=on
  Unit Delay : UnitDelay  SampleTime=-1  HasFrameUpgradeWarning=on
  filtered_val : Outport
  wires:
  MATLAB Function/1(filtered_val) -> filtered_val/1, Unit Delay/1
  raw_val/1 -> MATLAB Function/2(raw_val)
  Unit Delay/1 -> MATLAB Function/1(prev_val)
  freq_cut/1 -> MATLAB Function/3(freq_cut)

== system torch_pos_with_sensors_tuning(1)/POS_HOLD CONTROLLER/Vertical speed controller/Vertical position controller ==
  cur_alt : Inport
  tar_z : Inport  Port=2
  P_alt : Inport  Port=3
  Altitude PID : slpidlib/PID Controller  Controller=P  Form=Ideal  TimeDomain=Discrete-time  UseExternalTs=off  SampleTime=framePeriod_s  IntegratorMethod=Forward Euler  FilterMethod=Forward Euler  ControllerParametersSource=external  P=0  I=0  UseKiTs=off  D=0  UseExternalDerivativeSource=off  N=100  UseFilter=off  TunerSelectOption=Frequency Response Based  ZeroCross=off  InitialConditionSource=internal  InitialConditionForIntegrator=0  InitialConditionForFilter=0  DifferentiatorICPrevScaledInput=0  ExternalReset=either  TrackingMode=off  Kt=1  LimitOutput=on  SatLimitsSource=internal  UpperSaturationLimit=Aircraft.Control.v_z_max  LowerSaturationLimit=-Aircraft.Control.v_z_max  LinearizeAsGain=on  AntiWindupMode=clamping  Kb=1  LimitIntegrator=off  UpperIntegratorSaturationLimit=inf  LowerIntegratorSaturationLimit=-inf  POutMin=[]  POutMax=[]  IOutMin=[]  IOutMax=[]  DOutMin=[]  DOutMax=[]  NOutMin=[]  NOutMax=[]  SumOutMin=[]  SumOutMax=[]  SaturationOutMin=[]  SaturationOutMax=[]  PParamMin=[]  PParamMax=[]  IParamMin=[]  IParamMax=[]  DParamMin=[]  DParamMax=[]  NParamMin=[]  NParamMax=[]  KbParamMin=[]  KbParamMax=[]  KtParamMin=[]  KtParamMax=[]  KbOutMin=[]  KbOutMax=[]  KtOutMin=[]  KtOutMax=[]  IntegratorOutMin=[]  IntegratorOutMax=[]  FilterOutMin=[]  FilterOutMax=[]  SumI1OutMin=[]  SumI1OutMax=[]  SumI2OutMin=[]  SumI2OutMax=[]  SumI3OutMin=[]  SumI3OutMax=[]  SumI4OutMin=[]  SumI4OutMax=[]  SumDOutMin=[]  SumDOutMax=[]  DifferentiatorOutMin=[]  DifferentiatorOutMax=[]  FilterDiffOutCoefMin=[]  FilterDiffOutCoefMax=[]  ReciprocalOutMin=[]  ReciprocalOutMax=[]  SumDenOutMin=[]  SumDenOutMax=[]  SumNumOutMin=[]  SumNumOutMax=[]  DivideOutMin=[]  DivideOutMax=[]  UdiffTsProdOutMin=[]  UdiffTsProdOutMax=[]  NTsProdOutMin=[]  NTsProdOutMax=[]  UintegralTsProdOutMin=[]  UintegralTsProdOutMax=[]  UngainTsProdOutMin=[]  UngainTsProdOutMax=[]  ClampingZeroOutDataTypeStr=Inherit: Inherit via back propagation  ClampingZeroOutMin=[]  ClampingZeroOutMax=[]  FilterDenConstantOutDataTypeStr=Inherit: Inherit via back propagation  FilterDenConstantOutMin=[]  FilterDenConstantOutMax=[]  PCopyOutDataTypeStr=Inherit: Inherit via back propagation  PCopyOutMin=[]  PCopyOutMax=[]  NCopyOutDataTypeStr=Inherit: Inherit via back propagation  NCopyOutMin=[]  NCopyOutMax=[]  IntegratorContinuousStateAttributes=''  IntegratorStateMustResolveToSignalObject=off  IntegratorRTWStateStorageClass=Auto  FilterContinuousStateAttributes=''  FilterStateMustResolveToSignalObject=off  FilterRTWStateStorageClass=Auto  ParallelPVariant=ExternalParameters  IdealPVariant=Disabled  IVariant=Disabled  DVariant=Disabled  IntegratorVariant=Disabled  SatVariant=Enabled  AWVariant=Disabled  PCopyVariant=Disabled  TRVariant=Disabled  FdbkBlocksVariant=Forward  IdealPFdbkVariant=Disabled  SatFdbkVariant=Disabled  DerivativeFilterVariant=Disabled  NVariant=Disabled  NCopyVariant=Disabled_SignalSpec  FilterICVariant=Disabled  IntegratorICVariant=Disabled  ExternalResetVariant=Disabled  TRSumVariant=Passthrough  SumFdbkVariant=Disabled  SumVariant=Passthrough_P  TsampFilterVariant=InternalTs  TsampNgainVariant=Passthrough  TsampIntegralVariant=Disabled_SignalSpec  ExternalSaturationOutDataTypeStr=Inherit: Same as second input  DerivativeSourceVariant=Disabled
  Sum3 : Sum  Inputs=|+-
  ve_z_cmd_mps : Outport
  wires:
  Altitude PID/1 -> ve_z_cmd_mps/1
  tar_z/1 -> Sum3/1  "target_z"
  cur_alt/1 -> Sum3/2
  Sum3/1 -> Altitude PID/1
  P_alt/1 -> Altitude PID/2

== system torch_pos_with_sensors_tuning(1)/POS_HOLD CONTROLLER/Vertical speed controller/roll_D_DLPF ==
  raw_val : Inport
  freq_cut : Inport  Port=2
  Constant : Constant  Value=frameRate_hz  OutDataTypeStr=single
  MATLAB Function : MATLAB Function  TreatAsAtomicUnit=on
  Unit Delay : UnitDelay  SampleTime=-1  HasFrameUpgradeWarning=on
  filtered_val : Outport
  wires:
  freq_cut/1 -> MATLAB Function/3(freq_cut)
  MATLAB Function/1(filtered_val) -> Unit Delay/1, filtered_val/1
  Unit Delay/1 -> MATLAB Function/1(prev_val)
  raw_val/1 -> MATLAB Function/2(raw_val)
  Constant/1 -> MATLAB Function/4(samp_freq)

== system torch_pos_with_sensors_tuning(1)/POS_HOLD CONTROLLER/Vertical speed controller/set_tar_z when ve_z_cmd == 0 ==
  In1 : Inport
  Enable : EnablePort
  tar_z : Outport
  wires:
  In1/1 -> tar_z/1

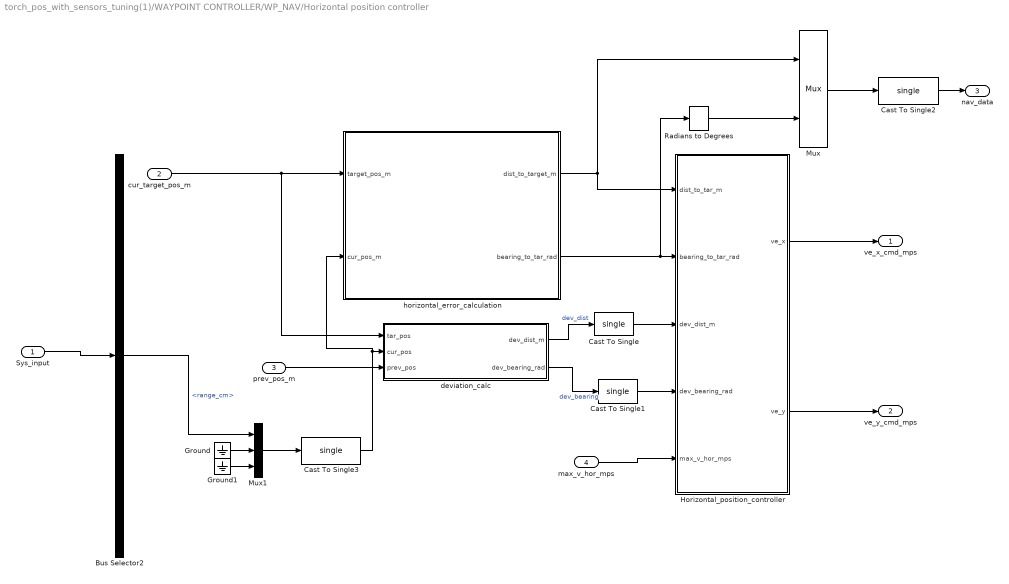
== system torch_pos_with_sensors_tuning(1)/WAYPOINT CONTROLLER/WP_NAV/Horizontal position controller ==
  Sys_input : Inport
  cur_target_pos_m : Inport  Port=2
  prev_pos_m : Inport  Port=3
  max_v_hor_mps : Inport  Port=4
  Bus Selector2 : BusSelector  OutputSignals=Sensor Data.tfmini.range_cm
  Cast To Single{,1..3} (4 alike) : DataTypeConversion  OutDataTypeStr=single  SaturateOnIntegerOverflow=off  RndMeth=Floor
  Ground : Ground
  Ground1 : Ground
  Horizontal_position_controller : Subsystem
  Mux : Mux  Inputs=2
  Mux1 : Mux  Inputs=3
  Radians to Degrees : simulink_extras/Transformations/Radians to Degrees
  deviation_calc : MATLAB Function  TreatAsAtomicUnit=on
  "horizontal_error_calculation " : Subsystem
  ve_x_cmd_mps : Outport
  ve_y_cmd_mps : Outport  Port=2
  nav_data : Outport  Port=3
  wires:
  Horizontal_position_controller/1(ve_x) -> ve_x_cmd_mps/1
  Horizontal_position_controller/2(ve_y) -> ve_y_cmd_mps/1
  Sys_input/1 -> Bus Selector2/1
  "horizontal_error_calculation "/1(dist_to_target_m) -> Horizontal_position_controller/1(dist_to_tar_m), Mux/1
  deviation_calc/1(dev_dist_m) -> Cast To Single/1  "dev_dist"
  cur_target_pos_m/1 -> deviation_calc/1(tar_pos), "horizontal_error_calculation "/1(target_pos_m)
  prev_pos_m/1 -> deviation_calc/3(prev_pos)
  max_v_hor_mps/1 -> Horizontal_position_controller/5(max_v_hor_mps)
  Cast To Single/1 -> Horizontal_position_controller/3(dev_dist_m)
  deviation_calc/2(dev_bearing_rad) -> Cast To Single1/1  "dev_bearing"
  Cast To Single1/1 -> Horizontal_position_controller/4(dev_bearing_rad)
  "horizontal_error_calculation "/2(bearing_to_tar_rad) -> Radians to Degrees/1, Horizontal_position_controller/2(bearing_to_tar_rad)
  Radians to Degrees/1 -> Mux/2
  Mux/1 -> Cast To Single2/1
  Cast To Single2/1 -> nav_data/1
  Bus Selector2/1 -> Mux1/1  "<range_cm>"
  Cast To Single3/1 -> "horizontal_error_calculation "/2(cur_pos_m), deviation_calc/2(cur_pos)
  Mux1/1 -> Cast To Single3/1
  Ground/1 -> Mux1/2
  Ground1/1 -> Mux1/3

== system torch_pos_with_sensors_tuning(1)/WAYPOINT CONTROLLER/WP_NAV/Subsystem ==
  Sys_input : Inport
  tar_pos : Inport  Port=2
  max_v_z_mps : Inport  Port=3
  Bus Selector : BusSelector  OutputSignals=Sensor Data.tfmini.range_cm
  Cast To Single : DataTypeConversion  OutDataTypeStr=single  SaturateOnIntegerOverflow=off  RndMeth=Floor
  Selector : Selector  InputPortWidth=3  IndexOptions=Index vector (dialog)  Indices=3  OutputSizes=1
  Vertical position controller1 : Subsystem
  ve_z_cmd_mps : Outport
  wires:
  Vertical position controller1/1(ve_z_cmd_mps) -> ve_z_cmd_mps/1  "ve_z_cmd_mps"
  tar_pos/1 -> Selector/1
  Sys_input/1 -> Bus Selector/1
  Bus Selector/1 -> Cast To Single/1  "<range_cm>"
  max_v_z_mps/1 -> Vertical position controller1/3(max_v_z_mps)
  Selector/1 -> Vertical position controller1/2(tar_z)
  Cast To Single/1 -> Vertical position controller1/1(cur_alt)

== system torch_pos_with_sensors_tuning(1)/WAYPOINT CONTROLLER/WP_NAV/Vertical position controller ==
  Sys_input : Inport
  max_v_z_mps : Inport  Port=2
  cur_target_pos_m : Inport  Port=3
  Bus Selector6 : BusSelector  OutputSignals=Navigation Filter Data.bfs_ekf.ned_pos_m
  Selector1 : Selector  InputPortWidth=3  IndexOptions=Index vector (dialog)  Indices=3  OutputSizes=1
  select_cur_z : Selector  InputPortWidth=3  IndexOptions=Index vector (dialog)  Indices=3  OutputSizes=1
  vertical_position_controller : Subsystem
  ve_z_cmd_mps : Outport
  wires:
  Sys_input/1 -> Bus Selector6/1
  Bus Selector6/1 -> select_cur_z/1  "<ned_pos_m>"
  vertical_position_controller/1(ve_z_cmd) -> ve_z_cmd_mps/1
  Selector1/1 -> vertical_position_controller/1(target_z_m)  "target_z"
  select_cur_z/1 -> vertical_position_controller/2(cur_z_m)
  cur_target_pos_m/1 -> Selector1/1
  max_v_z_mps/1 -> vertical_position_controller/3(max_v_z_mps)

== system torch_pos_with_sensors_tuning(1)/WAYPOINT CONTROLLER/WP_NAV/heading_controller ==
  Sys_input : Inport
  cur_target_heading_rad : Inport  Port=2
  Bus Selector4 : BusSelector  OutputSignals=Navigation Filter Data.bfs_ekf.heading_rad
  heading_controller : Subsystem
  yaw_rate_cmd_radps : Outport
  wires:
  Sys_input/1 -> Bus Selector4/1
  cur_target_heading_rad/1 -> heading_controller/1(heading_cmd_rad)
  Bus Selector4/1 -> heading_controller/2(<heading_rad>)  "<heading_rad>"
  heading_controller/1(yaw_rate_cmd) -> yaw_rate_cmd_radps/1

== system torch_pos_with_sensors_tuning(1)/determine arm and mode selection/Failsafe_management/Radio failsafe ==
  note: Transition to RTL mode
  note: If radio_failsafe is triggered and current_mode is not auto, rtl, land nor motor_state disarmed then RTL mode is triggered
  failsafe : Inport
  manual_mode : Inport  Port=2
  motor_state : Inport  Port=3
  AND1 : Logic  Commented=on  IconShape=distinctive  AllPortsSameDT=off  OutDataTypeStr=boolean
  Compare To Constant : simulink/Logic and Bit Operations/Compare To Constant  Commented=on  relop=~=  const=3  OutDataTypeStr=boolean
  Compare To Constant1 : simulink/Logic and Bit Operations/Compare To Constant  Commented=on  relop=~=  const=4  OutDataTypeStr=boolean
  Compare To Constant2 : simulink/Logic and Bit Operations/Compare To Constant  Commented=on  relop=~=  const=5  OutDataTypeStr=boolean
  NOR : Logic  Commented=on  Operator=NOR  Inputs=4  IconShape=distinctive  AllPortsSameDT=off  OutDataTypeStr=boolean
  NOT : Logic  Commented=on  Operator=NOT  IconShape=distinctive  AllPortsSameDT=off  OutDataTypeStr=boolean
  NOT1 : Logic  Operator=NOT  IconShape=distinctive  AllPortsSameDT=off  OutDataTypeStr=boolean
  Subsystem : Subsystem
  radio_failsafe_enabled : Outport
  wires:
  manual_mode/1 -> Compare To Constant2/1, Compare To Constant1/1, Compare To Constant/1
  Compare To Constant/1 -> NOR/1
  Compare To Constant1/1 -> NOR/2
  Compare To Constant2/1 -> NOR/3
  motor_state/1 -> NOT/1
  NOT/1 -> NOR/4
  failsafe/1 -> Subsystem/1(<inceptor_health>)
  NOR/1 -> AND1/1
  Subsystem/1(inceptor_health_filtered) -> NOT1/1
  NOT1/1 -> radio_failsafe_enabled/1

== system torch_pos_with_sensors_tuning(1)/determine arm and mode selection/Subsystem/e_stop counter ==
  note: This is to ensure e_stop event is not triggered unless e_stop command is sent for more than 0.3 s to prevent false trigger
  motor_e_stop_raw : Inport
  Enable : EnablePort  StatesWhenEnabling=reset
  Compare To Constant : simulink/Logic and Bit Operations/Compare To Constant  relop=>=  const=0.5  OutDataTypeStr=boolean
  Discrete-Time Integrator : DiscreteIntegrator  SampleTime=framePeriod_s  LimitOutput=on  UpperSaturationLimit=1  LowerSaturationLimit=0  ICPrevOutput=DiscIntNeverNeededParam  ICPrevScaledInput=DiscIntNeverNeededParam
  Gain : Gain  Gain=2
  e_stop_filtered : Outport
  wires:
  Compare To Constant/1 -> e_stop_filtered/1
  Discrete-Time Integrator/1 -> Compare To Constant/1
  Gain/1 -> Discrete-Time Integrator/1
  motor_e_stop_raw/1 -> Gain/1

== system torch_pos_with_sensors_tuning(1)/determine arm and mode selection/yaw_stick_arming/Enabled Subsystem ==
  yaw_input : Inport
  Enable : EnablePort  StatesWhenEnabling=reset
  Cast : DataTypeConversion  OutDataTypeStr=int8  SaturateOnIntegerOverflow=off  RndMeth=Floor
  Discrete-Time Integrator : DiscreteIntegrator  IntegratorMethod=Integration: Trapezoidal  SampleTime=framePeriod_s  OutDataTypeStr=single  UpperSaturationLimit=1  LowerSaturationLimit=0  ICPrevOutput=DiscIntNeverNeededParam  ICPrevScaledInput=DiscIntNeverNeededParam
  time_arm_valid_s : Outport
  wires:
  Discrete-Time Integrator/1 -> time_arm_valid_s/1
  Cast/1 -> Discrete-Time Integrator/1
  yaw_input/1 -> Cast/1

== system torch_pos_with_sensors_tuning(1)/determine arm and mode selection/yaw_stick_arming/manual_arming ==
  yaw_arm : Inport
  Trigger : TriggerPort  VariantControl=(inherit)  PortDimensions=1
  arm_state : Outport
  wires:
  yaw_arm/1 -> arm_state/1

== system torch_pos_with_sensors_tuning(1)/POS_HOLD CONTROLLER/Horizontal speed controller/Subsystem/roll_D_DLPF ==
  raw_val : Inport
  freq_cut : Inport  Port=2
  Constant : Constant  Value=50  OutDataTypeStr=single
  MATLAB Function : MATLAB Function  TreatAsAtomicUnit=on
  Unit Delay : UnitDelay  SampleTime=-1  HasFrameUpgradeWarning=on
  filtered_val : Outport
  wires:
  freq_cut/1 -> MATLAB Function/3(freq_cut)
  MATLAB Function/1(filtered_val) -> Unit Delay/1, filtered_val/1
  Unit Delay/1 -> MATLAB Function/1(prev_val)
  raw_val/1 -> MATLAB Function/2(raw_val)
  Constant/1 -> MATLAB Function/4(samp_freq)

== system torch_pos_with_sensors_tuning(1)/POS_HOLD CONTROLLER/Horizontal speed controller/zero_vel_handling/Horizontal position controller ==
  cur_target_pos_m : Inport
  cur_pos_m : Inport  Port=2
  Constant : Constant  Value=Aircraft.Control.P_v_hor
  Horizontal_position_controller : Subsystem
  "horizontal_error_calculation " : Subsystem
  ve_xy : Outport
  dist_to_tar : Outport  Port=2
  bearing_to_tar : Outport  Port=3
  wires:
  Horizontal_position_controller/1(Ve_xy) -> ve_xy/1
  "horizontal_error_calculation "/1(dist_to_target_m) -> dist_to_tar/1, Horizontal_position_controller/1(dist_to_tar_m)
  "horizontal_error_calculation "/2(bearing_to_tar_rad) -> bearing_to_tar/1, Horizontal_position_controller/2(bearing_to_tar_rad)
  cur_target_pos_m/1 -> "horizontal_error_calculation "/1(target_pos_m)
  cur_pos_m/1 -> "horizontal_error_calculation "/2(cur_pos_m)
  Constant/1 -> Horizontal_position_controller/3(gain)

== system torch_pos_with_sensors_tuning(1)/POS_HOLD CONTROLLER/Horizontal speed controller/zero_vel_handling/delay_on_instant_off ==
  in : Inport
  AND : Logic  IconShape=distinctive  AllPortsSameDT=off  OutDataTypeStr=boolean
  delayed : Subsystem
  out : Outport
  wires:
  delayed/1(delayed_sig) -> AND/1
  in/1 -> AND/2, delayed/1(sig)
  AND/1 -> out/1
